simulink model "LinearControl_sim"  (R2024b)
settings: Solver=VariableStepAuto  StartTime=0.0  StopTime=20  FixedStep=1e-6  MaxStep=1e-3  RelTol=1e-6  AbsTol=1e-4
values from neighbouring files (symbols this model uses):
  A = [ -1,       0,    -a*n*x_eq(3)^(n-1)/(1 + x_eq(3)^n)^2 ... (first row only)    [FBL.m]    (also in LinearControl.m; control.m)
  a = k^-3    (= 1000)    [Chapter2.m]    (also in FBL.m; LinearControl.m; SlidingMode.m; control.m)
  Ampdes = 2.2    [Chapter2.m]    (also in FBL.m; LinearControl.m; SlidingMode.m; control.m)
  Biasdes = 3.3    [Chapter2.m]    (also in FBL.m; LinearControl.m; SlidingMode.m; control.m)
  Freqdes = 2*pi/6    (= 1.0471975512)    [Chapter2.m]    (also in FBL.m; LinearControl.m; SlidingMode.m; control.m)
  Phasedes = 3*pi/2    (= 4.71238898038)    [Chapter2.m]    (also in FBL.m; LinearControl.m; SlidingMode.m; control.m)
  x_eq = fsolve(handle, x_0)    [Chapter2.m]    (also in DimensionalSystem.m = fsolve(handle, xi_0); FBL.m; LinearControl.m; SlidingMode.m)
libraries: slpidlib x2
settings Model: Creator=User  LastModifiedBy=robyr

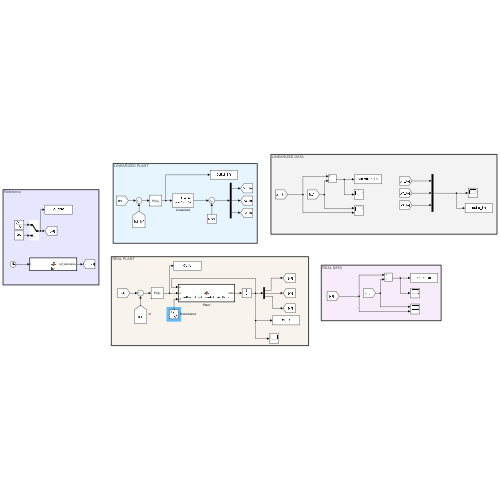
[thumbnail: Simulink's stored preview of the top-level diagram]
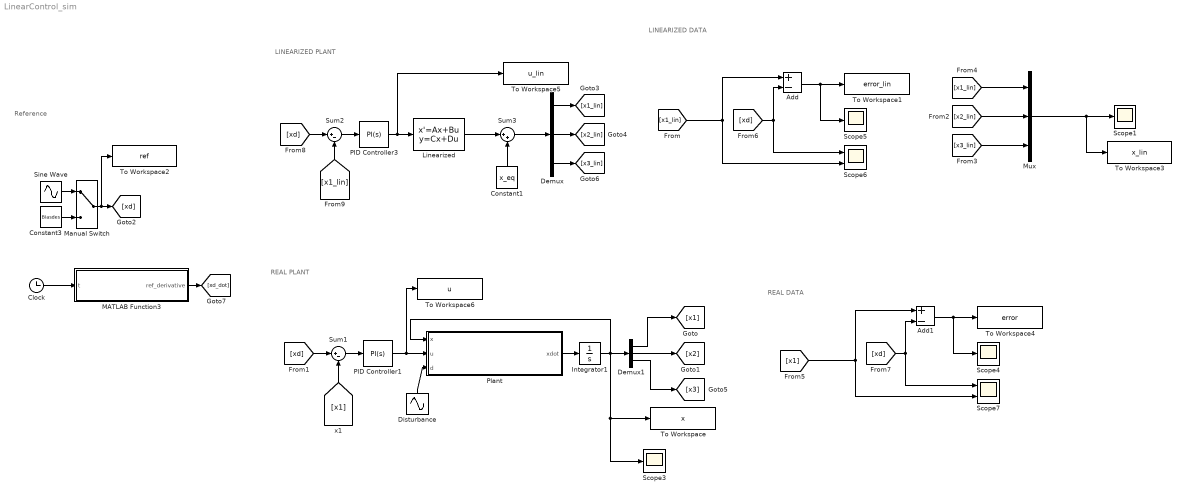
== system LinearControl_sim ==
  note: REAL PLANT
  note: Reference
  note: LINEARIZED PLANT
  note: LINEARIZED DATA
  note: REAL DATA
  Add : Sum  Inputs=+-
  Add1 : Sum  Inputs=+-
  Clock : Clock
  Constant1 : Constant  Value=x_eq
  Constant3 : Constant  Value=Biasdes
  Demux : Demux  Outputs=3
  Demux1 : Demux  Outputs=3
  Disturbance : Sin  Amplitude=0.2  Frequency=Freqdes*100  SampleTime=0
  Integrator1 : Integrator  InitialCondition=Biasdes *0.8*ones(3,1)
  Linearized : StateSpace  A=A  B=[a;0;0]  C=eye(3)  D=zeros(3,1)  InitialCondition=Biasdes *0.8*ones(3,1) - x_eq
  MATLAB Function3 : MATLAB Function  TreatAsAtomicUnit=on
  Manual Switch : ManualSwitch
  Mux : Mux  Inputs=3
  PID Controller1 : slpidlib/PID Controller  Controller=PI  Form=Parallel  TimeDomain=Continuous-time  UseExternalTs=off  SampleTime=-1  IntegratorMethod=Forward Euler  FilterMethod=Forward Euler  ControllerParametersSource=internal  P=0.015  I=0.01  UseKiTs=off  D=0.005  UseExternalDerivativeSource=off  N=100  UseFilter=on  TunerSelectOption=Transfer Function Based (PID Tuner App)  InitialConditionSource=internal  InitialConditionForIntegrator=0  InitialConditionForFilter=0  DifferentiatorICPrevScaledInput=0  ExternalReset=none  TrackingMode=off  Kt=1  LimitOutput=off  SatLimitsSource=internal  UpperSaturationLimit=inf  LowerSaturationLimit=-inf  LinearizeAsGain=on  AntiWindupMode=none  Kb=1  LimitIntegrator=off  UpperIntegratorSaturationLimit=inf  LowerIntegratorSaturationLimit=-inf  POutMin=[]  POutMax=[]  IOutMin=[]  IOutMax=[]  DOutMin=[]  DOutMax=[]  NOutMin=[]  NOutMax=[]  SumOutMin=[]  SumOutMax=[]  SaturationOutMin=[]  SaturationOutMax=[]  PParamMin=[]  PParamMax=[]  IParamMin=[]  IParamMax=[]  DParamMin=[]  DParamMax=[]  NParamMin=[]  NParamMax=[]  KbParamMin=[]  KbParamMax=[]  KtParamMin=[]  KtParamMax=[]  KbOutMin=[]  KbOutMax=[]  KtOutMin=[]  KtOutMax=[]  IntegratorOutMin=[]  IntegratorOutMax=[]  FilterOutMin=[]  FilterOutMax=[]  SumI1OutMin=[]  SumI1OutMax=[]  SumI2OutMin=[]  SumI2OutMax=[]  SumI3OutMin=[]  SumI3OutMax=[]  SumI4OutMin=[]  SumI4OutMax=[]  SumDOutMin=[]  SumDOutMax=[]  DifferentiatorOutMin=[]  DifferentiatorOutMax=[]  FilterDiffOutCoefMin=[]  FilterDiffOutCoefMax=[]  ReciprocalOutMin=[]  ReciprocalOutMax=[]  SumDenOutMin=[]  SumDenOutMax=[]  SumNumOutMin=[]  SumNumOutMax=[]  DivideOutMin=[]  DivideOutMax=[]  UdiffTsProdOutMin=[]  UdiffTsProdOutMax=[]  NTsProdOutMin=[]  NTsProdOutMax=[]  UintegralTsProdOutMin=[]  UintegralTsProdOutMax=[]  UngainTsProdOutMin=[]  UngainTsProdOutMax=[]  ClampingZeroOutDataTypeStr=Inherit: Inherit via back propagation  ClampingZeroOutMin=[]  ClampingZeroOutMax=[]  FilterDenConstantOutDataTypeStr=Inherit: Inherit via back propagation  FilterDenConstantOutMin=[]  FilterDenConstantOutMax=[]  PCopyOutDataTypeStr=Inherit: Inherit via back propagation  PCopyOutMin=[]  PCopyOutMax=[]  NCopyOutDataTypeStr=Inherit: Inherit via back propagation  NCopyOutMin=[]  NCopyOutMax=[]  IntegratorContinuousStateAttributes=''  IntegratorStateMustResolveToSignalObject=off  IntegratorRTWStateStorageClass=Auto  FilterContinuousStateAttributes=''  FilterStateMustResolveToSignalObject=off  FilterRTWStateStorageClass=Auto  ParallelPVariant=InternalParameters  IdealPVariant=Disabled  IVariant=InternalParameters  DVariant=Disabled  IntegratorVariant=Continuous  SatVariant=Disabled  AWVariant=Passthrough  PCopyVariant=Disabled  TRVariant=Disabled  FdbkBlocksVariant=Forward  IdealPFdbkVariant=Disabled  SatFdbkVariant=Disabled  DerivativeFilterVariant=Disabled  NVariant=Disabled  NCopyVariant=Disabled_SignalSpec  FilterICVariant=Disabled  IntegratorICVariant=InternalICs  ExternalResetVariant=Disabled  TRSumVariant=Passthrough  SumFdbkVariant=Disabled  SumVariant=Sum_PI  TsampFilterVariant=InternalTs  TsampNgainVariant=Passthrough  TsampIntegralVariant=Disabled_SignalSpec  ExternalSaturationOutDataTypeStr=Inherit: Same as second input  DerivativeSourceVariant=Disabled  PreIntVariant=InternalPreInt
  PID Controller3 : slpidlib/PID Controller  Controller=PI  Form=Parallel  TimeDomain=Continuous-time  UseExternalTs=off  SampleTime=-1  IntegratorMethod=Forward Euler  FilterMethod=Forward Euler  ControllerParametersSource=internal  P=0.015  I=0.01  UseKiTs=off  D=0.005  UseExternalDerivativeSource=off  N=100  UseFilter=on  TunerSelectOption=Transfer Function Based (PID Tuner App)  InitialConditionSource=internal  InitialConditionForIntegrator=0  InitialConditionForFilter=0  DifferentiatorICPrevScaledInput=0  ExternalReset=none  TrackingMode=off  Kt=1  LimitOutput=off  SatLimitsSource=internal  UpperSaturationLimit=inf  LowerSaturationLimit=-inf  LinearizeAsGain=on  AntiWindupMode=none  Kb=1  LimitIntegrator=off  UpperIntegratorSaturationLimit=inf  LowerIntegratorSaturationLimit=-inf  POutMin=[]  POutMax=[]  IOutMin=[]  IOutMax=[]  DOutMin=[]  DOutMax=[]  NOutMin=[]  NOutMax=[]  SumOutMin=[]  SumOutMax=[]  SaturationOutMin=[]  SaturationOutMax=[]  PParamMin=[]  PParamMax=[]  IParamMin=[]  IParamMax=[]  DParamMin=[]  DParamMax=[]  NParamMin=[]  NParamMax=[]  KbParamMin=[]  KbParamMax=[]  KtParamMin=[]  KtParamMax=[]  KbOutMin=[]  KbOutMax=[]  KtOutMin=[]  KtOutMax=[]  IntegratorOutMin=[]  IntegratorOutMax=[]  FilterOutMin=[]  FilterOutMax=[]  SumI1OutMin=[]  SumI1OutMax=[]  SumI2OutMin=[]  SumI2OutMax=[]  SumI3OutMin=[]  SumI3OutMax=[]  SumI4OutMin=[]  SumI4OutMax=[]  SumDOutMin=[]  SumDOutMax=[]  DifferentiatorOutMin=[]  DifferentiatorOutMax=[]  FilterDiffOutCoefMin=[]  FilterDiffOutCoefMax=[]  ReciprocalOutMin=[]  ReciprocalOutMax=[]  SumDenOutMin=[]  SumDenOutMax=[]  SumNumOutMin=[]  SumNumOutMax=[]  DivideOutMin=[]  DivideOutMax=[]  UdiffTsProdOutMin=[]  UdiffTsProdOutMax=[]  NTsProdOutMin=[]  NTsProdOutMax=[]  UintegralTsProdOutMin=[]  UintegralTsProdOutMax=[]  UngainTsProdOutMin=[]  UngainTsProdOutMax=[]  ClampingZeroOutDataTypeStr=Inherit: Inherit via back propagation  ClampingZeroOutMin=[]  ClampingZeroOutMax=[]  FilterDenConstantOutDataTypeStr=Inherit: Inherit via back propagation  FilterDenConstantOutMin=[]  FilterDenConstantOutMax=[]  PCopyOutDataTypeStr=Inherit: Inherit via back propagation  PCopyOutMin=[]  PCopyOutMax=[]  NCopyOutDataTypeStr=Inherit: Inherit via back propagation  NCopyOutMin=[]  NCopyOutMax=[]  IntegratorContinuousStateAttributes=''  IntegratorStateMustResolveToSignalObject=off  IntegratorRTWStateStorageClass=Auto  FilterContinuousStateAttributes=''  FilterStateMustResolveToSignalObject=off  FilterRTWStateStorageClass=Auto  ParallelPVariant=InternalParameters  IdealPVariant=Disabled  IVariant=InternalParameters  DVariant=Disabled  IntegratorVariant=Continuous  SatVariant=Disabled  AWVariant=Passthrough  PCopyVariant=Disabled  TRVariant=Disabled  FdbkBlocksVariant=Forward  IdealPFdbkVariant=Disabled  SatFdbkVariant=Disabled  DerivativeFilterVariant=Disabled  NVariant=Disabled  NCopyVariant=Disabled_SignalSpec  FilterICVariant=Disabled  IntegratorICVariant=InternalICs  ExternalResetVariant=Disabled  TRSumVariant=Passthrough  SumFdbkVariant=Disabled  SumVariant=Sum_PI  TsampFilterVariant=InternalTs  TsampNgainVariant=Passthrough  TsampIntegralVariant=Disabled_SignalSpec  ExternalSaturationOutDataTypeStr=Inherit: Same as second input  DerivativeSourceVariant=Disabled  PreIntVariant=InternalPreInt
  Plant : MATLAB Function  TreatAsAtomicUnit=on
  Scope{1,3..5} (4 alike) : Scope
  Scope6 : Scope  NumInputPorts=2
  Scope7 : Scope  NumInputPorts=2
  Sine Wave : Sin  Amplitude=Ampdes/10  Bias=Biasdes  Frequency=Freqdes  Phase=Phasedes  SampleTime=0
  Sum1 : Sum  Inputs=|+-
  Sum2 : Sum  Inputs=|+-
  Sum3 : Sum  Inputs=|++
  To Workspace : ToWorkspace  VariableName=x  SaveFormat=Timeseries  SampleTime=-1
  To Workspace1 : ToWorkspace  VariableName=error_lin  SaveFormat=Timeseries  SampleTime=-1
  To Workspace2 : ToWorkspace  VariableName=ref  SaveFormat=Timeseries  SampleTime=-1
  To Workspace3 : ToWorkspace  VariableName=x_lin  SaveFormat=Timeseries  SampleTime=-1
  To Workspace4 : ToWorkspace  VariableName=error  SaveFormat=Timeseries  SampleTime=-1
  To Workspace5 : ToWorkspace  VariableName=u_lin  SaveFormat=Timeseries  SampleTime=-1
  To Workspace6 : ToWorkspace  VariableName=u  SaveFormat=Timeseries  SampleTime=-1
  wires:
  Plant/1(xdot) -> Integrator1/1
  Integrator1/1 -> To Workspace/1, Scope3/1, Demux1/1, Plant/1(x)
  Add/1 -> Scope5/1, To Workspace1/1
  Demux1/1 -> [x1]
  Demux1/2 -> [x2]
  [x1_lin] -> Scope6/2, Add/1
  Demux1/3 -> [x3]
  [xd] -> Scope6/1, Add/2
  Sum1/1 -> PID Controller1/1
  Demux/1 -> [x1_lin]
  Demux/2 -> [x2_lin]
  Demux/3 -> [x3_lin]
  [x1] -> Sum1/2
  [x1_lin] -> Mux/1
  [x2_lin] -> Mux/2
  [x3_lin] -> Mux/3
  Mux/1 -> To Workspace3/1, Scope1/1
  Add1/1 -> Scope4/1, To Workspace4/1
  [x1] -> Scope7/2, Add1/1
  [xd] -> Scope7/1, Add1/2
  [xd] -> Sum1/1
  Manual Switch/1 -> To Workspace2/1, [xd]
  Clock/1 -> MATLAB Function3/1(t)
  MATLAB Function3/1(ref_derivative) -> [xd_dot]
  PID Controller1/1 -> To Workspace6/1, Plant/2(u)
  [xd] -> Sum2/1
  [x1_lin] -> Sum2/2
  Sum2/1 -> PID Controller3/1
  PID Controller3/1 -> To Workspace5/1, Linearized/1
  Linearized/1 -> Sum3/1
  Sum3/1 -> Demux/1
  Constant1/1 -> Sum3/2
  Sine Wave/1 -> Manual Switch/1
  Constant3/1 -> Manual Switch/2
  Disturbance/1 -> Plant/3(d)

== matlab function LinearControl_sim/MATLAB Function3 ==
  data: t input; ref_derivative output
function ref_derivative = fcn(t)

Ampdes=2.2/10 ;
Freqdes= 2*pi/6; 
Phasedes= 3*pi/2;


ref_derivative = Ampdes * Freqdes * cos(Freqdes * t + Phasedes);

== matlab function LinearControl_sim/Plant ==
  data: x input; u input; xdot output; d input
function xdot = adimensional_goodwin_oscillator(x,u,d)
b=0.1;
a=b^-3;
n=9;

xdot = [-x(1)+a/(1+x(3)^n) + a*u + d;...
        -x(2)+x(1);...
        -x(3)+ x(2);];
